simulink model "L9_tank_PID"  (Simulink 7.2)
settings: Solver=ode45  StartTime=0.0  StopTime=300  RelTol=1e-3
undefined symbols (not defined in the file or in its folder): G_PID_PAR, tank_pid
settings Model: Creator=kjartan  LastModifiedBy=kjartan  CovModelRefEnable=off
settings DataIOCC: SaveFormat=StructureWithTime
settings OptimizationCC: ExpressionDepthLimit=128
settings DebuggingCC: UnderspecifiedInitializationDetection=Simplified  MergeDetectMultiDrivingBlocksExec=error  SolverPrmCheckMsg=none  FcnCallInpInsideContextMsg=Enable All  StateNameClashWarn=none  StrictBusMsg=ErrorLevel1
settings HardwareCC: ProdIntDivRoundTo=Zero  ProdEndianess=LittleEndian  ProdHWDeviceType=Specified
settings CodeAppCC: CustomSymbolStrType=$N$R$M_T
settings GRTTargetCC: TargetFunctionLibrary=C89/C90 (ANSI)

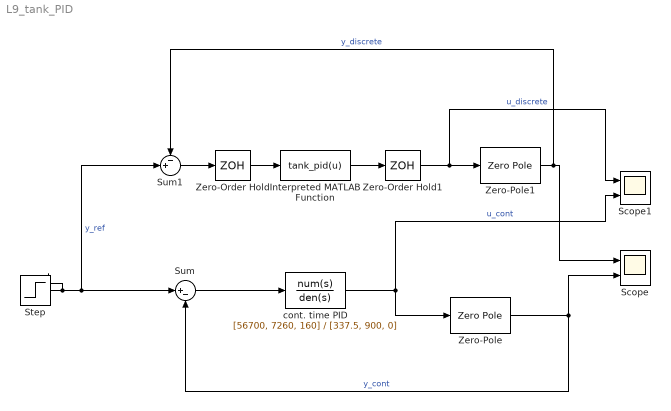
== system L9_tank_PID ==
  Interpreted MATLAB Function : MATLABFcn  MATLABFcn=tank_pid(u)  OutputDimensions=1
  Scope : Scope  NumInputPorts=2
      settings: TimeRange=auto  MaxDataPoints=5000  SaveToWorkspace=off  SaveName=ScopeData  YMin=-0.22125~-5  YMax=1.98198~5  SampleTime=-1
  Scope1 : Scope  NumInputPorts=2
      settings: TimeRange=auto  MaxDataPoints=5000  SaveToWorkspace=off  YMin=-27.54216~-5  YMax=189.72691~5  SampleTime=-1
  Step : Step  SampleTime=0
  Sum : Sum  Inputs=|+-
  Sum1 : Sum  Inputs=-+|
  Zero-Order Hold : ZeroOrderHold  SampleTime=G_PID_PAR.h
  Zero-Order Hold1 : ZeroOrderHold  SampleTime=G_PID_PAR.h
  Zero-Pole : ZeroPole  Zeros=[]  Poles=[-0.0179, -0.0129]  Gain=[0.00048]
  Zero-Pole1 : ZeroPole  Zeros=[]  Poles=[-0.0179, -0.0129]  Gain=[0.00048]
  cont. time PID : TransferFcn  Numerator=[56700, 7260, 160]  Denominator=[337.5, 900, 0]
  wires:
  Sum/1 -> cont. time PID/1
  Zero-Pole/1 -> Scope/2, Sum/2  "y_cont"
  Step/1 -> Sum1/2, Sum/1  "y_ref"
  Zero-Order Hold/1 -> Interpreted MATLAB Function/1
  Interpreted MATLAB Function/1 -> Zero-Order Hold1/1
  Zero-Order Hold1/1 -> Scope1/1, Zero-Pole1/1  "u_discrete"
  cont. time PID/1 -> Scope1/2, Zero-Pole/1  "u_cont"
  Zero-Pole1/1 -> Scope/1, Sum1/1  "y_discrete"
  Sum1/1 -> Zero-Order Hold/1
